simulink model "mppt"  (R2024b)
settings: Solver=VariableStepAuto  StartTime=0.0  StopTime=1  RelTol=1e-3
libraries: spsSeriesRLCBranchLib x4, spsDCVoltageSourceLib x1, spsDiodeLib x1, spsIGBTDiodeLib x1, spsPVArrayLib x1, eePwmGenerator x1, spsVoltageMeasurementLib x1, sps_lib x1
settings Model: Creator=User  LastModifiedBy=User

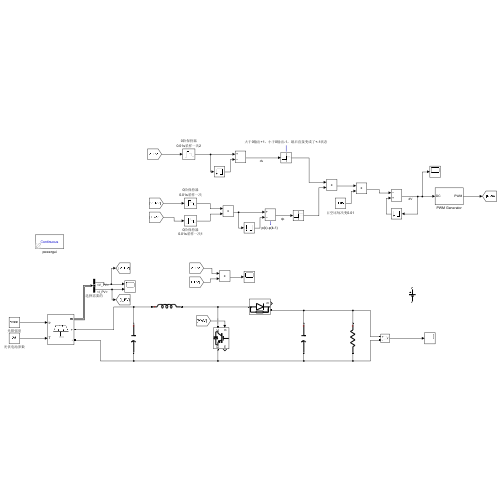
[thumbnail: Simulink's stored preview of the top-level diagram]
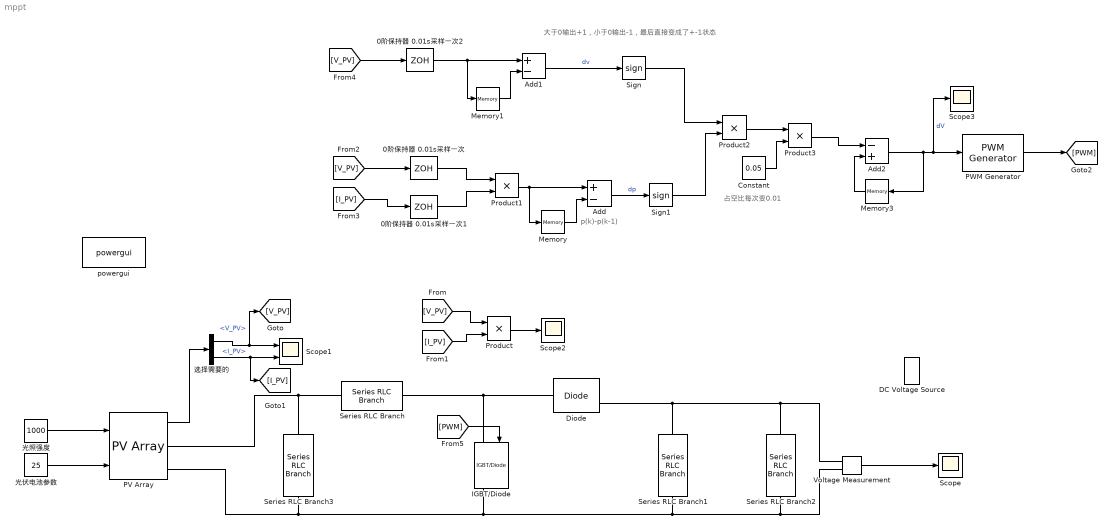
== system mppt ==
  note: 占空比每次变0.01
  note: 大于0输出+1，小于0输出-1，最后直接变成了+-1状态
  note: p(k)-p(k-1)
  0阶保持器 0.01s采样一次 : ZeroOrderHold  SampleTime=0.01
  0阶保持器 0.01s采样一次1 : ZeroOrderHold  SampleTime=0.01
  0阶保持器 0.01s采样一次2 : ZeroOrderHold  SampleTime=0.01
  Add : Sum  Inputs=+-
  Add1 : Sum  Inputs=+-
  Add2 : Sum  Inputs=-+
  Constant : Constant  Value=0.05
  DC Voltage Source : spsDCVoltageSourceLib/DC Voltage Source  Amplitude=29  Measurements=None
  Diode : spsDiodeLib/Diode  Ron=0.001  Lon=0  Vf=0.8  IC=0  UseSnubber=0  Rs=500  Cs=250e-9  Measurements=on
  IGBT/Diode : spsIGBTDiodeLib/IGBT//Diode  Ron=1e-3  Rs=1e5  Cs=inf  Measurements=on
  Memory : Memory
  Memory1 : Memory
  Memory3 : Memory
  PV Array : spsPVArrayLib/PV Array  Npar=5  Nser=1  PlotType=array @ 25 deg.C & specified irradiances  S_vec="[ 1000  500  100 ]"  Temp_C_vec="[ 45 25  ]"  ModuleName=User-defined  PlotWhenSelected=off  Pm=213.15  Ncell=60  Voc=36.3  Isc=7.84  Vm=29  Im=7.35  beta_Voc_pc=-0.36099  alpha_Isc_pc=0.102  beta_Voc=-0.13104  alpha_Isc=0.0079968  IL=7.8654  I0=2.9273e-10  nI=0.98119  Rsh=313.0553  Rs=0.39381  RobustModel=off  RobustCellTemperature=313.3991  BAL=on  Tc=1e-6  Tfilter=5e-5
  PWM Generator : eePwmGenerator/PWM Generator  CarrCount=Up  Tper=1e3  Tdelay=0  Ts=0
  Product{,1..3} (4 alike) : Product
  Scope : Scope
  Scope1 : Scope  NumInputPorts=2
  Scope2 : Scope
  Scope3 : Scope
  Series RLC Branch : spsSeriesRLCBranchLib/Series RLC Branch  LConnTagsString=__new0  RConnTagsString=__new0  BranchType=L  Resistance=1  Inductance=1e-2  SetiL0=off  InitialCurrent=0  Capacitance=1e-6  Setx0=off  InitialVoltage=0  Measurements=None
  Series RLC Branch1 : spsSeriesRLCBranchLib/Series RLC Branch  LConnTagsString=__new0  RConnTagsString=__new0  BranchType=C  Resistance=1  Inductance=1e-3  SetiL0=off  InitialCurrent=0  Capacitance=1e-2  Setx0=off  InitialVoltage=0  Measurements=None
  Series RLC Branch2 : spsSeriesRLCBranchLib/Series RLC Branch  LConnTagsString=__new0  RConnTagsString=__new0  BranchType=R  Resistance=1  Inductance=1e-3  SetiL0=off  InitialCurrent=0  Capacitance=1e-6  Setx0=off  InitialVoltage=0  Measurements=None
  Series RLC Branch3 : spsSeriesRLCBranchLib/Series RLC Branch  LConnTagsString=__new0  RConnTagsString=__new0  BranchType=C  Resistance=1  Inductance=1e-3  SetiL0=off  InitialCurrent=0  Capacitance=1e-3  Setx0=off  InitialVoltage=0  Measurements=None
  Sign : Signum
  Sign1 : Signum
  Voltage Measurement : spsVoltageMeasurementLib/Voltage Measurement  PhasorSimulation=off  OutputType=Complex  PSBequivalent=0
  powergui : sps_lib/powergui  Priority=1  SimulationMode=Continuous  SampleTime=50e-6  frequency=60  Iterations=50  frequencyindice=0  Pbase=100e6  ErrMax=1e-4  UnitsV=kV  UnitsW=MW  buscounter=0  FunctionMessages=off  echomessages=off  EnableUseOfTLC=off  CurrentSourceSwitches=off  DisableSnubberDevices=off  DisableRonSwitches=off  DisableVfSwitches=off  DisplayEquations=off  AutomaticDiscreteSolvers=off  SolverType=Tustin/Backward Euler (TBE)  Interpol=off  ExternalGateDelay=off  methode=off  Ts=100  x0status=blocks  SPID=on  SwTol=0  HookPort=off  NonlinearTolerance=1e-4  nMaxIteration=100  ContinueOnMaxIteration=off  RestoreLinks=warning  ResistiveCurrentMeasurement=off  Frange=[0:2:500]  Ylog=off  Xlog=on  ShowGrid=off  save=off  variable=ZData  structure=0  ZoomFFT=off  StartTime=0.0  cycles=1  DisplayStyle=1  fundamental=60  FreqAxis=off  MaxFrequency=1000  frequencyindicesteady=1  RmsSteady=1  display=off
  光伏电池参数 : Constant  Value=25
  光照强度 : Constant  Value=1000
  选择需要的 : BusSelector  OutputSignals=V_PV,I_PV
  wires:
  Voltage Measurement/1 -> Scope/1
  光照强度/1 -> PV Array/1
  光伏电池参数/1 -> PV Array/2
  PV Array/1 -> 选择需要的/1
  选择需要的/1 -> [V_PV], Scope1/1  "<V_PV>"
  选择需要的/2 -> [I_PV], Scope1/2  "<I_PV>"
  [V_PV] -> Product/1
  [I_PV] -> Product/2
  Product/1 -> Scope2/1
  Product1/1 -> Memory/1, Add/1
  [V_PV] -> 0阶保持器 0.01s采样一次/1
  0阶保持器 0.01s采样一次/1 -> Product1/1
  [I_PV] -> 0阶保持器 0.01s采样一次1/1
  0阶保持器 0.01s采样一次1/1 -> Product1/2
  Memory/1 -> Add/2
  Add/1 -> Sign1/1  "dp"
  [V_PV] -> 0阶保持器 0.01s采样一次2/1
  0阶保持器 0.01s采样一次2/1 -> Memory1/1, Add1/1
  Memory1/1 -> Add1/2
  Add1/1 -> Sign/1  "dv"
  Sign1/1 -> Product2/2
  Sign/1 -> Product2/1
  Product2/1 -> Product3/1
  Constant/1 -> Product3/2
  Product3/1 -> Add2/1
  Memory3/1 -> Add2/2
  Add2/1 -> Memory3/1, Scope3/1, PWM Generator/1  "dV"
  PWM Generator/1 -> [PWM]
  [PWM] -> IGBT/Diode/1
  connections:
  Diode/LConn1 -- IGBT/Diode/LConn1 -- Series RLC Branch/RConn1
  Diode/RConn1 -- Series RLC Branch2/LConn1 -- Voltage Measurement/LConn1 -- Series RLC Branch1/LConn1
  Series RLC Branch1/RConn1 -- PV Array/RConn2 -- Series RLC Branch3/RConn1 -- IGBT/Diode/RConn1 -- Voltage Measurement/LConn2 -- Series RLC Branch2/RConn1
  Series RLC Branch/LConn1 -- Series RLC Branch3/LConn1 -- PV Array/RConn1
